simulink model "propulsion_sim_thermo_simulink"  (R2026b)
settings: Solver=VariableStepAuto
undefined symbols (not defined in the file or in its folder): DiscIntNeverNeededParam
settings Model: Creator=taeta  LastModifiedBy=thoma
settings RTWCC: GPUComputeCapability=5.0

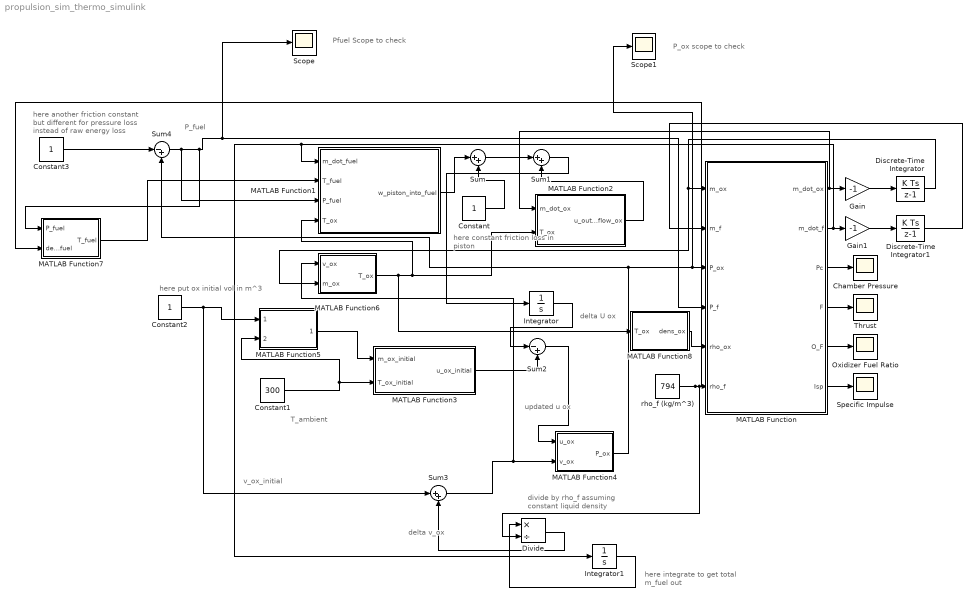
== system propulsion_sim_thermo_simulink ==
  note: P_ox scope to check
  note: Pfuel Scope to check
  note: P_fuel
  note: here another friction constant
      |
      |
      |
      |
      | but different for
      | pressure loss instead of raw
      | energy loss
  note: delta v_ox
  note: divide by rho_f assuming
      | constant liquid density
  note: here integrate to get total
      | m_fuel out
  note: v_ox_initial
  note: here put ox initial vol
      | in m^3
  note: T_ambient
  note: updated
      | u ox
  note: delta U ox
  note: here constant
      | friction loss in piston
  Chamber Pressure : Scope
      settings: ActiveDisplayYMinimum=-1  ActiveDisplayYMaximum=1
  Constant : Constant
  Constant1 : Constant  Value=300
  Constant2 : Constant
  Constant3 : Constant
  Discrete-Time Integrator : DiscreteIntegrator  InitialCondition=33.8916  SampleTime=-1  ICPrevOutput=DiscIntNeverNeededParam  ICPrevScaledInput=DiscIntNeverNeededParam
  Discrete-Time Integrator1 : DiscreteIntegrator  InitialCondition=9.678  SampleTime=-1  ICPrevOutput=DiscIntNeverNeededParam  ICPrevScaledInput=DiscIntNeverNeededParam
  Divide : Product  Inputs=*/
  Gain : Gain  Gain=-1
  Gain1 : Gain  Gain=-1
  Integrator : Integrator
  Integrator1 : Integrator
  MATLAB Function : MATLAB Function  TreatAsAtomicUnit=on
  MATLAB Function1 : MATLAB Function  TreatAsAtomicUnit=on
  MATLAB Function2 : MATLAB Function  TreatAsAtomicUnit=on
  MATLAB Function3 : MATLAB Function  TreatAsAtomicUnit=on
  MATLAB Function4 : MATLAB Function  TreatAsAtomicUnit=on
  MATLAB Function5 : MATLAB Function  TreatAsAtomicUnit=on
  MATLAB Function6 : MATLAB Function  TreatAsAtomicUnit=on
  MATLAB Function7 : MATLAB Function  TreatAsAtomicUnit=on
  MATLAB Function8 : MATLAB Function  TreatAsAtomicUnit=on
  Oxidizer Fuel Ratio : Scope
      settings: ActiveDisplayYMinimum=-1  ActiveDisplayYMaximum=1  DataLoggingVariableName=ScopeData2
  Scope : Scope
      settings: DataLoggingVariableName=ScopeData4
  Scope1 : Scope
      settings: DataLoggingVariableName=ScopeData5
  Specific Impulse : Scope
      settings: ActiveDisplayYMinimum=-1  ActiveDisplayYMaximum=1  DataLoggingVariableName=ScopeData3
  Sum : Sum  Inputs=|++
  Sum1 : Sum  Inputs=|++
  Sum2 : Sum  Inputs=|-+
  Sum3 : Sum  Inputs=|++
  Sum4 : Sum  Inputs=|-+
  Thrust : Scope
      settings: ActiveDisplayYMinimum=-1  ActiveDisplayYMaximum=1
  rho_f (kg/m^3) : Constant  Value=794
  wires:
  MATLAB Function/2(m_dot_f) -> Integrator1/1, MATLAB Function1/1(m_dot_fuel), Gain1/1
  Discrete-Time Integrator/1 -> MATLAB Function6/2(m_ox), MATLAB Function/1(m_ox)
  Discrete-Time Integrator1/1 -> MATLAB Function/2(m_f)
  Gain/1 -> Discrete-Time Integrator/1
  Gain1/1 -> Discrete-Time Integrator1/1
  MATLAB Function8/1(dens_ox) -> MATLAB Function/5(rho_ox)
  MATLAB Function/6(Isp) -> Specific Impulse/1
  MATLAB Function/5(O_F) -> Oxidizer Fuel Ratio/1
  MATLAB Function/4(F) -> Thrust/1
  MATLAB Function/3(Pc) -> Chamber Pressure/1
  MATLAB Function1/1(w_piston_into_fuel) -> Sum/1
  Constant/1 -> Sum/2
  Sum/1 -> Sum1/1
  Integrator/1 -> Sum2/1
  MATLAB Function3/1(u_ox_initial) -> Sum2/2
  Sum2/1 -> MATLAB Function4/1(u_ox)
  Constant1/1 -> MATLAB Function5/2(T_ox_initial), MATLAB Function3/2(T_ox_initial)
  Constant2/1 -> Sum3/1, MATLAB Function5/1(v_ox_initial)
  MATLAB Function5/1(m_ox_initial) -> MATLAB Function3/1(m_ox_initial)
  MATLAB Function/1(m_dot_ox) -> MATLAB Function2/1(m_dot_ox), Gain/1
  rho_f (kg/m^3)/1 -> MATLAB Function7/2(dens_fuel), Divide/2, MATLAB Function/6(rho_f)
  Integrator1/1 -> Divide/1
  Divide/1 -> Sum3/2
  Sum3/1 -> MATLAB Function6/1(v_ox), MATLAB Function4/2(v_ox)
  MATLAB Function4/1(P_ox) -> Scope1/1, MATLAB Function/3(P_ox), Sum4/2
  Sum1/1 -> Integrator/1
  MATLAB Function2/1(u_out_per_s_from_flow_ox) -> Sum1/2
  Constant3/1 -> Sum4/1
  Sum4/1 -> MATLAB Function1/3(P_fuel), MATLAB Function7/1(P_fuel), Scope/1, MATLAB Function/4(P_f)
  MATLAB Function7/1(T_fuel) -> MATLAB Function1/2(T_fuel)
  MATLAB Function6/1(T_ox) -> MATLAB Function8/1(T_ox), MATLAB Function1/4(T_ox), MATLAB Function2/2(T_ox)

== matlab function propulsion_sim_thermo_simulink/MATLAB Function1 ==
  data: m_dot_fuel input; w_piston_into_fuel output; T_fuel input; P_fuel input; T_ox input
function w_piston_into_fuel = fcn(m_dot_fuel,T_fuel,P_fuel,T_ox)

vchange_fuel_per_s=m_dot_fuel/py.CoolProp.CoolProp.PropsSI('D', 'T', T_fuel,'P',P_fuel,'Ethanol');
w_piston_into_fuel=vchange_fuel_per_s*py.CoolProp.CoolProp.PropsSI('P', 'T', T_ox, 'Q', 0, 'N2O');
%%%% gives work of piston received by fuel

== matlab function propulsion_sim_thermo_simulink/MATLAB Function ==
  data: m_ox input; m_dot_ox output; m_f input; P_ox input; P_f input; rho_ox input; rho_f input; m_dot_f output; Pc output; F output; O_F output; Isp output
function [m_dot_ox, m_dot_f, Pc, F, O_F, Isp] = engine_solver(m_ox, m_f, P_ox, P_f, rho_ox, rho_f)

    % output dimensions for simulink (everything equals 0 at first)
    m_dot_ox = 0;
    m_dot_f = 0;
    Pc = 0;
    F = 0;
    O_F = 0;
    Isp = 0;

    % constants
    g0 = 9.81; % m/s^2
    c_star = 2639.4; % m/s
    A_t = 7.85398e-5; % m^2
    A_e = 1.8816e-3; % m^2
    C_f = A_e / A_t; % thrust coefficient

    % initial guesses [m_dot_ox (kg/s); m_dot_f (kg/s); Pc (Pa)]
    x0 = [1.66337; 0.478249; 435.113 * 6894.76];

    % optimization for simulink or else it wont work
    options = optimoptions('fsolve', ...
        'Algorithm', 'levenberg-marquardt', ...
        'Display', 'off', ...
        'FunctionTolerance', 1e-6);

    % solve non-linear residual system
    [x_sol, ~, exitflag] = fsolve(@(x) engine_residuals(x, P_ox, P_f, rho_ox, rho_f, A_t, c_star), x0, options);

    if exitflag <= 0
        x_sol = x0; % so if solver fails to converge it like fixes itself basiaclly
    end

    % gets the solved state values
    m_dot_ox = abs(x_sol(1));
    m_dot_f = abs(x_sol(2));
    Pc = abs(x_sol(3));

    % engine performance outputs
    m_dot_tot = m_dot_ox + m_dot_f;
    F = C_f * Pc * A_t;
    O_F = m_dot_ox / max(m_dot_f, 1e-6);
    Isp = F / (max(m_dot_tot, 1e-6) * g0);
end

function R = engine_residuals(x, P_ox, P_f, rho_ox, rho_f, A_t, c_star)
    m_dot_ox_guess = abs(x(1));
    m_dot_f_guess = abs(x(2));
    Pc_guess = abs(x(3));

    % line losses using oxidizer and fuel constants
    dp_ox = calculate_line_loss_ox(m_dot_ox_guess, rho_ox);
    dp_f = calculate_line_loss_f(m_dot_f_guess, rho_f);

    % residual equations (assuming we want R=0)
    R_ox = P_ox - dp_ox - Pc_guess;
    R_f = P_f - dp_f - Pc_guess;
    R_c = (m_dot_ox_guess + m_dot_f_guess) - (Pc_guess * A_t / c_star);

    R = [R_ox; R_f; R_c];

    % this is so NaN/inf doesnt happen to fsolve
    if any(~isfinite(R))
        R = [1e6; 1e6; 1e6];
    end
end

function dp = calculate_line_loss_ox(m_dot, rho)
    % oxidizer line parameters
    g0 = 9.81;
    rho_safe = max(rho, 1e-3);
    
    f = 0.04; % friction factor
    D = 0.0535088; % pipe diameter (m)
    L = 0.762; % pipe length (m)
    k = 10; % minor loss coefficient
    Cv = 9; % valve flow coefficient
    A_inj = 2.20893e-5; % injector area (m^2)
    dz = 0.9144; % elevation change (m)
    
    % velocity and dynamic pressur
    A_pipe = (pi / 4) * D^2;
    v = m_dot / (rho_safe * A_pipe);
    q = 0.5 * rho_safe * (v^2);

    % individual pressure loss terms
    dp_pipe = f * (L / D) * q; % pipe loss
    dp_k = k * q; % minor loss
    
    % valve loss: i made it so that it converts m_dot to GPM for Cv equation
    SG = rho_safe / 1000; % specific gravity
    Q_gpm = (m_dot / rho_safe) * 15850.32; % m^3/s to GPM
    dp_v = SG * (Q_gpm / Cv)^2 * 6894.76; % converted psi to Pa
    
    dp_inj = 0.5 * (m_dot / A_inj)^2 / rho_safe; % injector loss
    dp_g = rho_safe * g0 * dz; % hydrostatic loss

    % total oxidizer pressure drop (Pa)
    dp = dp_pipe + dp_k + dp_v + dp_inj + dp_g;
end

function dp = calculate_line_loss_f(m_dot, rho)
    % fuel fine parameters
    g0 = 9.81;
    rho_safe = max(rho, 1e-3);
    f = 0.04; % friction factor
    D = 0.01270; % pipe diameter (m)
    L = 0.762; % pipe length (m)
    k = 10; % minor loss coefficient
    Cv = 5.228; % valve flow coefficient
    A_inj = 1.8816e-3; % injector area (m^2)
    dz= 0.9144; % elevation change (m)

    % velocity and dynamics pressue
    A_pipe = (pi / 4) * D^2;
    v = m_dot / (rho_safe * A_pipe);
    q = 0.5 * rho_safe * (v^2);

    % individual pressure loss terms
    dp_pipe = f * (L / D) * q;
    dp_k = k * q;
    
    SG = rho_safe / 1000;
    Q_gpm = (m_dot / rho_safe) * 15850.32;
    dp_v = SG * (Q_gpm / Cv)^2 * 6894.76;
    
    dp_inj = 0.5 * (m_dot / A_inj)^2 / rho_safe;
    dp_g = rho_safe * g0 * dz;

    % total fuel pressure drop (Pa)
    dp = dp_pipe + dp_k + dp_v + dp_inj + dp_g;
end

== matlab function propulsion_sim_thermo_simulink/MATLAB Function2 ==
  data: m_dot_ox input; u_out_per_s_from_flow_ox output; T_ox input
function u_out_per_s_from_flow_ox = fcn(m_dot_ox,T_ox)

u_out_per_s_from_flow_ox=m_dot_ox*py.CoolProp.CoolProp.PropsSI('U', 'T', T_ox, 'Q', 0,'N2O');

== matlab function propulsion_sim_thermo_simulink/MATLAB Function3 ==
  data: m_ox_initial input; u_ox_initial output; T_ox_initial input
function u_ox_initial = fcn(m_ox_initial,T_ox_initial)

u_ox=m_ox*py.CoolProp.CoolProp.PropsSI('U', 'T', T_ox,'Q',0,'N2O');
%%%gives original u of oxidizer

== matlab function propulsion_sim_thermo_simulink/MATLAB Function4 ==
  data: u_ox input; P_ox output; v_ox input
function P_ox = fcn(u_ox, v_ox)

== matlab function propulsion_sim_thermo_simulink/MATLAB Function5 ==
  data: v_ox_initial input; m_ox_initial output; T_ox_initial input
function m_ox_initial = fcn(v_ox_initial,T_ox_initial)

m_ox_initial=v_ox_initial*py.CoolProp.CoolProp.PropsSI('D', 'T', T_ox_initial, 'Q', 0, 'N2O');

== matlab function propulsion_sim_thermo_simulink/MATLAB Function6 ==
  data: v_ox input; T_ox output; m_ox input
function T_ox = fcn(v_ox,m_ox)

T_ox=py.CoolProp.CoolProp.PropsSI('T','D',(m_ox/v_ox),'Q', 0, 'N2O');

== matlab function propulsion_sim_thermo_simulink/MATLAB Function7 ==
  data: P_fuel input; T_fuel output; dens_fuel input
function T_fuel = fcn(P_fuel,dens_fuel)

T_fuel=py.CoolProp.CoolProp.PropsSI('T', 'D',dens_fuel,'P',P_fuel,'Ethanol');

== matlab function propulsion_sim_thermo_simulink/MATLAB Function8 ==
  data: T_ox input; dens_ox output
function dens_ox = fcn(T_ox)


dens_ox=py.CoolProp.CoolProp.PropsSI('D', 'T', T_ox, 'Q', 0, 'N2O');
